simulink model "DTMF"  (Simulink 8.7)
settings: Solver=FixedStepDiscrete  SolverMode=SingleTasking  StartTime=0.0  StopTime=5.5  RelTol=1e-3
PreLoadFcn:
  | load dspafxr;
libraries: dspstat3 x9, dspsrcs4 x8
settings Model: Creator=sv7  LastModifiedBy=Student
settings SolverCC: PositivePriorityOrder=on
settings DataIOCC: LimitDataPoints=off  SignalLoggingSaveFormat=ModelDataLogs  SaveOutput=off  SaveTime=off
settings OptimizationCC: DefaultParameterBehavior=Inlined  InlineInvariantSignals=on  ExpressionDepthLimit=2147483647  InitFltsAndDblsToZero=on  OptimizeModelRefInitCode=on  LifeSpan=1
settings DebuggingCC: SaveWithParameterizedLinksMsg=none  SignalResolutionControl=TryResolveAllWithWarning  SolverPrmCheckMsg=warning  MultiTaskDSMMsg=warning  MultiTaskCondExecSysMsg=none  FcnCallInpInsideContextMsg=UseLocalSettings  StateNameClashWarn=warning
settings HardwareCC: ProdBitPerLong=40  ProdLargestAtomicInteger=Integer  ProdIntDivRoundTo=Zero  ProdEndianess=LittleEndian  ProdHWDeviceType=Texas Instruments->C6000  TargetBitPerLong=40  TargetLargestAtomicInteger=Integer  TargetIntDivRoundTo=Zero  TargetEndianess=LittleEndian  TargetHWDeviceType=TI C6000
settings RTWCC: SystemTargetFile=idelink_ert.tlc  GenerateMakefile=off  TemplateMakefile=none  Description=IDE Link ERT
settings CodeAppCC: IgnoreCustomStorageClasses=off
settings TargetCC: CompOptLevelCompliant=off  ConcurrentExecutionCompliant=on  CombineOutputUpdateFcns=on  ERTFirstTimeCompliant=on  ERTCustomFileBanners=on  SupportContinuousTime=off  MATLABClassNameForMDSCustomization=linkfoundation.pjtgenerator.IdelinkCustomization  ModelStepFunctionPrototypeControlCompliant=on  GRTInterface=off
settings CustomProperty: DataType=string
settings TargetHardwareResources: Description=Target Hardware Resources Component
settings MATStruct: boardType=C6713DSK  isSimulator=[0.0]  enableHSRTDX=[0.0]  versionNumber=3.0  enableDSPBIOSTab=[0.0]  RTOS=DSP/BIOS  peripherals=[]  procName=CPU_1  boardName=C6713 DSK  realtimesupport=on  tag=ccslinktgtpref_ccsv5  deviceID=C6713  subFamily=671x  cpuClockRateMHz=[225.0]  codegenhookpoint=C6000  mvSwitch=-mv6710  numSections=[13.0]  numRTOS=[2.0]  defaultSysStackSize=[8192.0]  isBuiltIn=[1.0]  numBanks=[1.0]  numCacheLvl=[1.0]  isremovable=[0.0]  iscontentsfixed=[0.0]  name=IRAM  addr=[0.0]  size=[262144.0]  contents=Code & Data  space=Internal  createHeap=[0.0]  heapSize=[256.0]  defineLabel=[0.0]  heapLabel=segment_name  label=L2  timer=[]  timerprescaler=[]  description=C code  codeObjectMem=SDRAM  dataObjectMem=SDRAM  levelLabel=L2  cacheSize=64 kb  enable=off  schedulerType=Rate priority  schedulingMode=real-time  baseRatePriority=[7.0]  stackSize=[4096.0]  staticStackMemSegment=IRAM  dynamicStackMemSegment=SDRAM  errId=[]

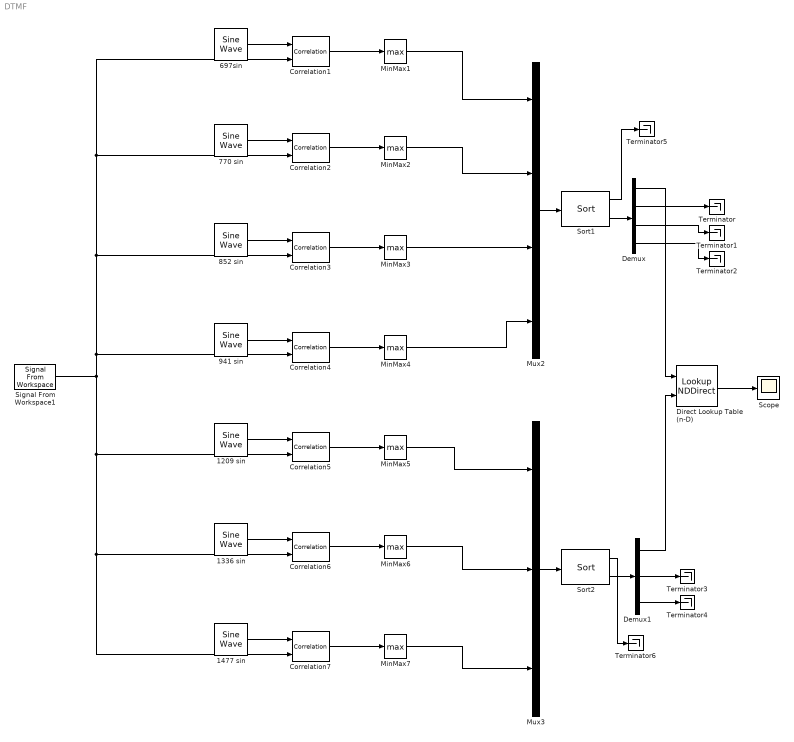
== system DTMF ==
  1209 sin : dspsrcs4/Sine Wave  Amplitude=1  Frequency=1209  Phase=0  SampleMode=Discrete  OutComplex=Real  CompMethod=Trigonometric fcn  TableSize=Speed  SampleTime=1/8000  SamplesPerFrame=40  ResetState=Restart at time zero  OutputFrames=on  dataType=double  wordLen=16  udDataType=sfix(16)  fracBitsMode=Best precision  numFracBits=15  OutDataTypeStr=double  LastOutDataTypeStr=double
  1336 sin : dspsrcs4/Sine Wave  Amplitude=1  Frequency=1336  Phase=0  SampleMode=Discrete  OutComplex=Real  CompMethod=Trigonometric fcn  TableSize=Speed  SampleTime=1/8000  SamplesPerFrame=40  ResetState=Restart at time zero  OutputFrames=on  dataType=double  wordLen=16  udDataType=sfix(16)  fracBitsMode=Best precision  numFracBits=15  OutDataTypeStr=double  LastOutDataTypeStr=double
  1477 sin : dspsrcs4/Sine Wave  Amplitude=1  Frequency=1477  Phase=0  SampleMode=Discrete  OutComplex=Real  CompMethod=Trigonometric fcn  TableSize=Speed  SampleTime=1/8000  SamplesPerFrame=40  ResetState=Restart at time zero  OutputFrames=on  dataType=double  wordLen=16  udDataType=sfix(16)  fracBitsMode=Best precision  numFracBits=15  OutDataTypeStr=double  LastOutDataTypeStr=double
  697sin : dspsrcs4/Sine Wave  Amplitude=1  Frequency=697  Phase=0  SampleMode=Discrete  OutComplex=Real  CompMethod=Trigonometric fcn  TableSize=Speed  SampleTime=1/8000  SamplesPerFrame=40  ResetState=Restart at time zero  OutputFrames=on  dataType=double  wordLen=16  udDataType=sfix(16)  fracBitsMode=Best precision  numFracBits=15  OutDataTypeStr=double  LastOutDataTypeStr=double
  770 sin : dspsrcs4/Sine Wave  Amplitude=1  Frequency=770  Phase=0  SampleMode=Discrete  OutComplex=Real  CompMethod=Trigonometric fcn  TableSize=Speed  SampleTime=1/8000  SamplesPerFrame=40  ResetState=Restart at time zero  OutputFrames=on  dataType=double  wordLen=16  udDataType=sfix(16)  fracBitsMode=Best precision  numFracBits=15  OutDataTypeStr=double  LastOutDataTypeStr=double
  852 sin : dspsrcs4/Sine Wave  Amplitude=1  Frequency=852  Phase=0  SampleMode=Discrete  OutComplex=Real  CompMethod=Trigonometric fcn  TableSize=Speed  SampleTime=1/8000  SamplesPerFrame=40  ResetState=Restart at time zero  OutputFrames=on  dataType=double  wordLen=16  udDataType=sfix(16)  fracBitsMode=Best precision  numFracBits=15  OutDataTypeStr=double  LastOutDataTypeStr=double
  941 sin : dspsrcs4/Sine Wave  Amplitude=1  Frequency=941  Phase=0  SampleMode=Discrete  OutComplex=Real  CompMethod=Trigonometric fcn  TableSize=Speed  SampleTime=1/8000  SamplesPerFrame=40  ResetState=Restart at time zero  OutputFrames=on  dataType=double  wordLen=16  udDataType=sfix(16)  fracBitsMode=Best precision  numFracBits=15  OutDataTypeStr=double  LastOutDataTypeStr=double
  Correlation{1..7} (7 alike) : dspstat3/Correlation  domain=Time  outputDataTypeStr=Inherit: Same as accumulator  outputLastDataTypeStr=Inherit: Same as accumulator  outputMin=[]  outputMax=[]  roundingMode=Floor  overflowMode=off
  Demux : Demux
  Demux1 : Demux  Outputs=3
  Direct Lookup Table (n-D) : LookupNDDirect  Table=[0 0 0 0;0 1 2 3; 0 4 5 6; 0 7 8 9; 0 0 0 0]
  MinMax{1..7} (7 alike) : MinMax  Function=max
  Mux2 : Mux
  Mux3 : Mux  Inputs=3
  Scope : Scope
  Signal From Workspace1 : dspsrcs4/Signal From Workspace  X=PhoneNum  Ts=1/8000  nsamps=40  OutputAfterFinalValue=Cyclic repetition  ignoreOrWarnInputAndFrameLengths=off  OutputFrames=on
  Sort1 : dspstat3/Sort  otype=Value and Index  dir=Descending  sortAlg=Quick sort  accumDataTypeStr=Inherit: Same as product output  accumLastDataTypeStr=Inherit: Same as product output  roundingMode=Floor  overflowMode=off
  Sort2 : dspstat3/Sort  otype=Value and Index  dir=Descending  sortAlg=Quick sort  accumDataTypeStr=Inherit: Same as product output  accumLastDataTypeStr=Inherit: Same as product output  roundingMode=Floor  overflowMode=off
  Terminator{,1..6} (7 alike) : Terminator
  wires:
  MinMax2/1 -> Mux2/2
  MinMax3/1 -> Mux2/3
  941 sin/1 -> Correlation4/1
  Correlation4/1 -> MinMax4/1
  Correlation5/1 -> MinMax5/1
  Correlation2/1 -> MinMax2/1
  MinMax4/1 -> Mux2/4
  1336 sin/1 -> Correlation6/1
  852 sin/1 -> Correlation3/1
  MinMax1/1 -> Mux2/1
  Correlation1/1 -> MinMax1/1
  Correlation3/1 -> MinMax3/1
  770 sin/1 -> Correlation2/1
  697sin/1 -> Correlation1/1
  Mux2/1 -> Sort1/1
  MinMax5/1 -> Mux3/1
  1209 sin/1 -> Correlation5/1
  Correlation6/1 -> MinMax6/1
  MinMax6/1 -> Mux3/2
  Mux3/1 -> Sort2/1
  MinMax7/1 -> Mux3/3
  Correlation7/1 -> MinMax7/1
  1477 sin/1 -> Correlation7/1
  Sort1/2 -> Demux/1
  Demux/1 -> Direct Lookup Table (n-D)/1
  Demux1/1 -> Direct Lookup Table (n-D)/2
  Sort2/2 -> Demux1/1
  Signal From Workspace1/1 -> Correlation4/2, Correlation3/2, Correlation1/2, Correlation2/2, Correlation5/2, Correlation6/2, Correlation7/2
  Demux/2 -> Terminator/1
  Demux/3 -> Terminator1/1
  Demux/4 -> Terminator2/1
  Demux1/3 -> Terminator4/1
  Demux1/2 -> Terminator3/1
  Sort1/1 -> Terminator5/1
  Sort2/1 -> Terminator6/1
  Direct Lookup Table (n-D)/1 -> Scope/1
